simulink model "samv71_Xplained_Ultra_Standalone"  (R2020b)
settings: Solver=FixedStepDiscrete  StartTime=0.0  StopTime=1  FixedStep=0.001  RelTol=1e-3  EnableMultiTasking=on
undefined symbols (not defined in the file or in its folder): LQFP144, PA21, PA24, PA25, PB0, PB1, PB2, PB3, PB4, PD28, PD30, Pin, SAMV71Q21B, Timer
libraries: MCHP_Blockset x19, simulink x5
(part 2 of 2)

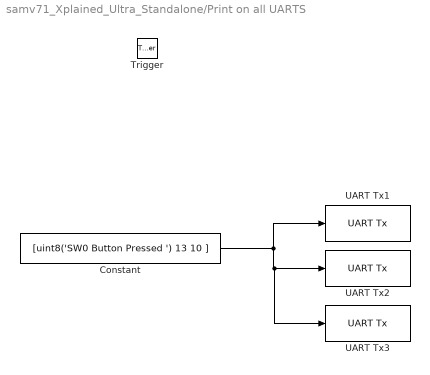
== system samv71_Xplained_Ultra_Standalone/Print on all UARTS ==
  Trigger : TriggerPort  VariantControl=Variant  PortDimensions=1
  Constant : Constant  Value=[uint8('SW0 Button Pressed ') 13 10 ]  OutDataTypeStr=uint8  SampleTime=-1
  UART Tx1 : MCHP_Blockset/BUS UART/UART Tx  UART_REF=USART 1  ORDERING=None  AllOrNothing=off  SampleTime=-1  MCHP_MASTERLINK=samv71_Xplained_Ultra_Standalone/Microchip Master  NSend_Input=off  UART_String=off  NSend_Output=off
      settings: SourceProductName=MPLAB Device Blocks for Simulink
  UART Tx2 : MCHP_Blockset/BUS UART/UART Tx  UART_REF=USART 0  ORDERING=None  AllOrNothing=off  SampleTime=-1  MCHP_MASTERLINK=samv71_Xplained_Ultra_Standalone/Microchip Master  NSend_Input=off  UART_String=off  NSend_Output=off
      settings: SourceProductName=MPLAB Device Blocks for Simulink
  UART Tx3 : MCHP_Blockset/BUS UART/UART Tx  UART_REF=UART 3  ORDERING=None  AllOrNothing=off  SampleTime=-1  MCHP_MASTERLINK=samv71_Xplained_Ultra_Standalone/Microchip Master  NSend_Input=off  UART_String=off  NSend_Output=off
      settings: SourceProductName=MPLAB Device Blocks for Simulink
  wires:
  Constant/1 -> UART Tx3/1, UART Tx2/1, UART Tx1/1

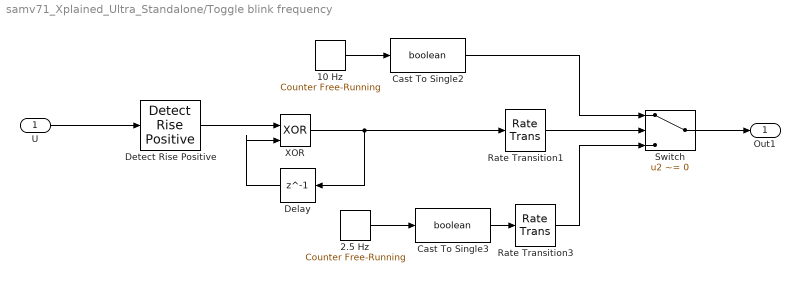
== system samv71_Xplained_Ultra_Standalone/Toggle blink frequency ==
  U : Inport
  10 Hz : simulink/Sources/Counter Free-Running  NumBits=1  tsamp=0.05
  2.5 Hz : simulink/Sources/Counter Free-Running  NumBits=1  tsamp=0.2
  Cast To Single2 : DataTypeConversion  OutDataTypeStr=boolean
  Cast To Single3 : DataTypeConversion  OutDataTypeStr=boolean
  Delay : Delay  DelayLength=1  InitialCondition=0
  Detect Rise Positive : simulink/Logic and Bit Operations/Detect Rise Positive  vinit=0  OutDataTypeStr=boolean
  Rate Transition1 : RateTransition
  Rate Transition3 : RateTransition
  Switch : Switch  Criteria=u2 ~= 0
  XOR : Logic  Operator=XOR  IconShape=distinctive  AllPortsSameDT=off  OutDataTypeStr=boolean
  Out1 : Outport
  wires:
  XOR/1 -> Rate Transition1/1, Delay/1
  Cast To Single2/1 -> Switch/1
  Cast To Single3/1 -> Rate Transition3/1
  Rate Transition1/1 -> Switch/2
  10 Hz/1 -> Cast To Single2/1
  Detect Rise Positive/1 -> XOR/1
  Switch/1 -> Out1/1
  Delay/1 -> XOR/2
  2.5 Hz/1 -> Cast To Single3/1
  U/1 -> Detect Rise Positive/1
  Rate Transition3/1 -> Switch/3
